simulink model "slau2"  (Simulink 9.1)
settings: Solver=ode45  StartTime=0.0  StopTime=5.0  RelTol=1e-3  EnableMultiTasking=on
settings Model: Creator=pustovskix.2018  LastModifiedBy=bukova.2018
settings DataIOCC: LimitDataPoints=on  SignalLoggingSaveFormat=ModelDataLogs
settings OptimizationCC: ExpressionDepthLimit=2147483647
settings DebuggingCC: SolverPrmCheckMsg=warning  FcnCallInpInsideContextMsg=warning  StateNameClashWarn=warning
settings GRTTargetCC: GeneratePreprocessorConditionals=Disable all

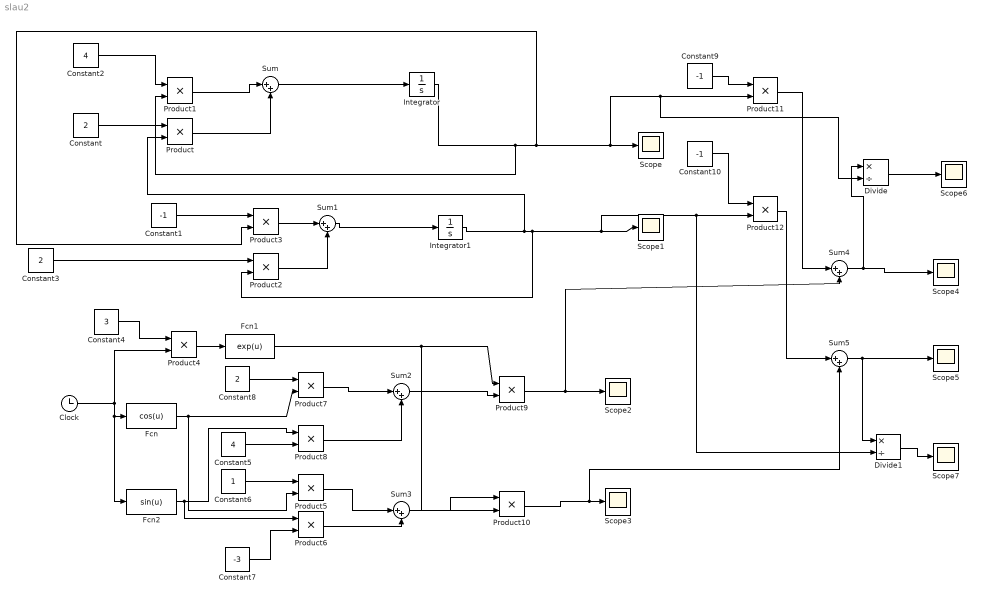
== system slau2 ==
  Clock : Clock
  Constant : Constant  Value=2
  Constant1 : Constant  Value=-1
  Constant10 : Constant  Value=-1
  Constant2 : Constant  Value=4
  Constant3 : Constant  Value=2
  Constant4 : Constant  Value=3
  Constant5 : Constant  Value=4
  Constant6 : Constant
  Constant7 : Constant  Value=-3
  Constant8 : Constant  Value=2
  Constant9 : Constant  Value=-1
  Divide : Product  Inputs=*/
  Divide1 : Product  Inputs=*/
  Fcn : Fcn  Expr=cos(u)
  Fcn1 : Fcn  Expr=exp(u)
  Fcn2 : Fcn  Expr=sin(u)
  Integrator : Integrator  InitialCondition=2
  Integrator1 : Integrator  InitialCondition=1
  Product{,1..12} (13 alike) : Product  RndMeth=Zero
  Scope{,1..7} (8 alike) : Scope
  Sum{,1..5} (6 alike) : Sum  Inputs=|++
  wires:
  Integrator1/1 -> Product2/2, Scope1/1, Divide1/2, Product12/2, Product/2
  Integrator/1 -> Product3/2, Scope/1, Divide/2, Product11/2, Product1/2
  Sum/1 -> Integrator/1
  Sum1/1 -> Integrator1/1
  Constant3/1 -> Product2/1
  Constant1/1 -> Product3/1
  Constant2/1 -> Product1/1
  Constant/1 -> Product/1
  Product1/1 -> Sum/1
  Product/1 -> Sum/2
  Product3/1 -> Sum1/1
  Product2/1 -> Sum1/2
  Clock/1 -> Fcn2/1, Fcn/1, Product4/2
  Constant4/1 -> Product4/1
  Product4/1 -> Fcn1/1
  Constant7/1 -> Product6/2
  Constant6/1 -> Product5/1
  Constant5/1 -> Product8/2
  Constant8/1 -> Product7/1
  Fcn/1 -> Product7/2, Product5/2
  Fcn2/1 -> Product8/1, Product6/1
  Product6/1 -> Sum3/2
  Product5/1 -> Sum3/1
  Product7/1 -> Sum2/1
  Product8/1 -> Sum2/2
  Fcn1/1 -> Product9/1, Product10/2
  Sum3/1 -> Product10/1
  Sum2/1 -> Product9/2
  Product9/1 -> Scope2/1, Sum4/2
  Product10/1 -> Scope3/1, Sum5/2
  Constant10/1 -> Product12/1
  Constant9/1 -> Product11/1
  Product11/1 -> Sum4/1
  Product12/1 -> Sum5/1
  Sum5/1 -> Divide1/1, Scope5/1
  Sum4/1 -> Divide/1, Scope4/1
  Divide/1 -> Scope6/1
  Divide1/1 -> Scope7/1
